simulink model "discreate_control_by_period"  (R2015a)
settings: Solver=ode45  StartTime=0.0  StopTime=10  RelTol=1e-3
values from neighbouring files (symbols this model uses):
  Cs = Kp * (Ti*s + 1) / (Ti*s)    [main.m]
  Gs = 3 / (6*s + 1)    [main.m]
  h = 0.12 + 0.012 * i    [main.m]
settings Model: Creator=Steven  LastModifiedBy=Xiaotian

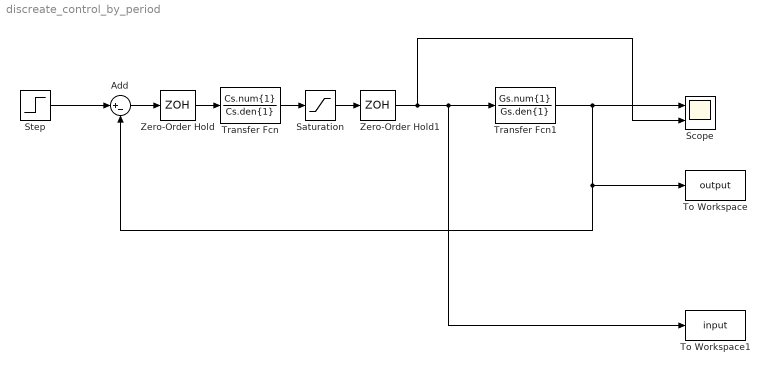
== system discreate_control_by_period ==
  Add : Sum  Inputs=|+-
  Saturation : Saturate  UpperLimit=12  LowerLimit=-12
  Scope : Scope  NumInputPorts=2
      settings: TimeRange=20  YMin=-8~-15  YMax=10~15
  Step : Step  Time=0  SampleTime=0
  To Workspace : ToWorkspace  VariableName=output  SaveFormat=Timeseries  SampleTime=h
  To Workspace1 : ToWorkspace  VariableName=input  SaveFormat=Timeseries  SampleTime=h
  Transfer Fcn : TransferFcn  Numerator=Cs.num{1}  Denominator=Cs.den{1}
  Transfer Fcn1 : TransferFcn  Numerator=Gs.num{1}  Denominator=Gs.den{1}
  Zero-Order Hold : ZeroOrderHold  SampleTime=h
  Zero-Order Hold1 : ZeroOrderHold  SampleTime=h
  wires:
  Zero-Order Hold/1 -> Transfer Fcn/1
  Add/1 -> Zero-Order Hold/1
  Transfer Fcn1/1 -> Scope/1, To Workspace/1, Add/2
  Zero-Order Hold1/1 -> To Workspace1/1, Transfer Fcn1/1, Scope/2
  Step/1 -> Add/1
  Transfer Fcn/1 -> Saturation/1
  Saturation/1 -> Zero-Order Hold1/1
